simulink subsystem "PowerSystemRef"  (R2024b)
settings: Solver=VariableStepAuto  StartTime=0.0  StopTime=10.0  RelTol=1e-3
undefined symbols (not defined in the file): ess, geom, mot, mot2, mot3, mot4, propel, propel2, propel3, propel4, pxf_diagram_options, SimIn, tc, tc2, tc3, tc4
libraries: simulink x10, slpidlib x5
(part 5 of 10)

== system PowerSystemRef/powerplant/mot4/ctrl/cmd ==
  inport-main_info_bus-1 : Inport
  aInport--2 : Inport  Port=2
  aInport--3 : Inport  Port=3
  aInport--4 : Inport  Port=4
  Terminator_1 : Terminator
  Terminator_2 : Terminator
  Terminator_3 : Terminator
  mot4_ctrl_cmd_map_Pelec_funTW_volt_in : Subsystem
  parameter_out : Subsystem
  parameter_selection : Subsystem
  outport-system_info_bus : Outport
  wires:
  inport-main_info_bus-1/1 -> parameter_selection/1(inport-main_info_bus-1)
  parameter_out/1(outport-system_info_bus) -> outport-system_info_bus/1
  mot4_ctrl_cmd_map_Pelec_funTW_volt_in/1(mot_ctrl_cmd_simu) -> parameter_out/1(inport-mot4_ctrl_cmd_simu)
  parameter_selection/1(outport-mot4_plant_spd_out_simu-1) -> mot4_ctrl_cmd_map_Pelec_funTW_volt_in/1(mot_plant_spd_out_simu)
  parameter_selection/2(outport-mot4_ctrl_trs_trq_simu-2) -> mot4_ctrl_cmd_map_Pelec_funTW_volt_in/2(mot_ctrl_trs_trq_simu)
  parameter_selection/3(outport-mot4_ctrl_cstr_trq_max_pos_simu-3) -> mot4_ctrl_cmd_map_Pelec_funTW_volt_in/3(mot_ctrl_cstr_trq_max_pos_simu)
  parameter_selection/4(outport-mot4_ctrl_cstr_trq_max_neg_simu-4) -> mot4_ctrl_cmd_map_Pelec_funTW_volt_in/4(mot_ctrl_cstr_trq_max_neg_simu)
  aInport--2/1 -> Terminator_1/1
  aInport--3/1 -> Terminator_2/1
  aInport--4/1 -> Terminator_3/1

== system PowerSystemRef/powerplant/mot4/ctrl/cstr ==
  inport-main_info_bus-1 : Inport
  aInport--2 : Inport  Port=2
  aInport--3 : Inport  Port=3
  Terminator_1 : Terminator
  Terminator_2 : Terminator
  mot4_ctrl_cstr_map_Pelec_funTW_volt_in : Subsystem
  parameter_out : Subsystem
  parameter_selection : Subsystem
  outport-system_info_bus : Outport
  outport-cstr_bus : Outport  Port=2
  wires:
  inport-main_info_bus-1/1 -> parameter_selection/1(inport-main_info_bus-1)
  parameter_out/1(outport-system_info_bus) -> outport-system_info_bus/1
  parameter_out/2(outport-cstr_bus) -> outport-cstr_bus/1
  mot4_ctrl_cstr_map_Pelec_funTW_volt_in/1(mot_ctrl_cstr_trq_pk_pos_simu) -> parameter_out/1(inport-mot4_ctrl_cstr_trq_pk_pos_simu)
  mot4_ctrl_cstr_map_Pelec_funTW_volt_in/2(mot_ctrl_cstr_trq_max_pos_simu) -> parameter_out/2(inport-mot4_ctrl_cstr_trq_max_pos_simu)
  mot4_ctrl_cstr_map_Pelec_funTW_volt_in/3(mot_ctrl_cstr_trq_pk_neg_simu) -> parameter_out/3(inport-mot4_ctrl_cstr_trq_pk_neg_simu)
  mot4_ctrl_cstr_map_Pelec_funTW_volt_in/4(mot_ctrl_cstr_trq_max_neg_simu) -> parameter_out/4(inport-mot4_ctrl_cstr_trq_max_neg_simu)
  mot4_ctrl_cstr_map_Pelec_funTW_volt_in/5(mot_ctrl_cstr_trq_cont_pos_simu) -> parameter_out/5(inport-mot4_ctrl_cstr_trq_cont_pos_simu)
  mot4_ctrl_cstr_map_Pelec_funTW_volt_in/6(mot_ctrl_cstr_trq_cont_neg_simu) -> parameter_out/6(inport-mot4_ctrl_cstr_trq_cont_neg_simu)
  mot4_ctrl_cstr_map_Pelec_funTW_volt_in/7(mot_ctrl_cstr_temp_coeff_simu) -> parameter_out/7(inport-mot4_ctrl_cstr_temp_coeff_simu)
  parameter_selection/1(outport-mot4_plant_spd_out_simu-1) -> mot4_ctrl_cstr_map_Pelec_funTW_volt_in/1(mot_plant_spd_out_simu)
  parameter_selection/2(outport-mot4_plant_temp_coeff_simu-2) -> mot4_ctrl_cstr_map_Pelec_funTW_volt_in/2(mot_plant_temp_coeff_simu)
  aInport--2/1 -> Terminator_1/1
  aInport--3/1 -> Terminator_2/1

== system PowerSystemRef/powerplant/mot4/ctrl/dmd ==
  inport-main_info_bus-1 : Inport
  aInport--2 : Inport  Port=2
  Terminator_1 : Terminator
  mot4_ctrl_dmd_uas : Subsystem
  parameter_out : Subsystem
  parameter_selection : Subsystem
  outport-system_info_bus : Outport
  outport-dmd_bus : Outport  Port=2
  wires:
  inport-main_info_bus-1/1 -> parameter_selection/1(inport-main_info_bus-1)
  parameter_out/1(outport-system_info_bus) -> outport-system_info_bus/1
  parameter_out/2(outport-dmd_bus) -> outport-dmd_bus/1
  mot4_ctrl_dmd_uas/1(mot_ctrl_trs_trq_simu) -> parameter_out/1(inport-mot4_ctrl_trs_trq_simu)
  mot4_ctrl_dmd_uas/2(mot_ctrl_ratedpwr_simu) -> parameter_out/2(inport-mot4_ctrl_ratedpwr_simu)
  parameter_selection/1(outport-apc_ctrl_dt4_simu-1) -> mot4_ctrl_dmd_uas/1(apc_ctrl_dt_simu)
  parameter_selection/2(outport-env_plant_density_simu-2) -> mot4_ctrl_dmd_uas/2(env_plant_density_simu)
  parameter_selection/3(outport-ess_ctrl_pwr_max_pro_simu-3) -> mot4_ctrl_dmd_uas/3(ess_ctrl_pwr_max_pro_simu)
  parameter_selection/4(outport-propel4_plant_speed_simu-4) -> mot4_ctrl_dmd_uas/4(propel_plant_speed_simu)
  parameter_selection/5(outport-tc4_plant_spd_in_simu-5) -> mot4_ctrl_dmd_uas/5(tc_plant_spd_in_simu)
  aInport--2/1 -> Terminator_1/1

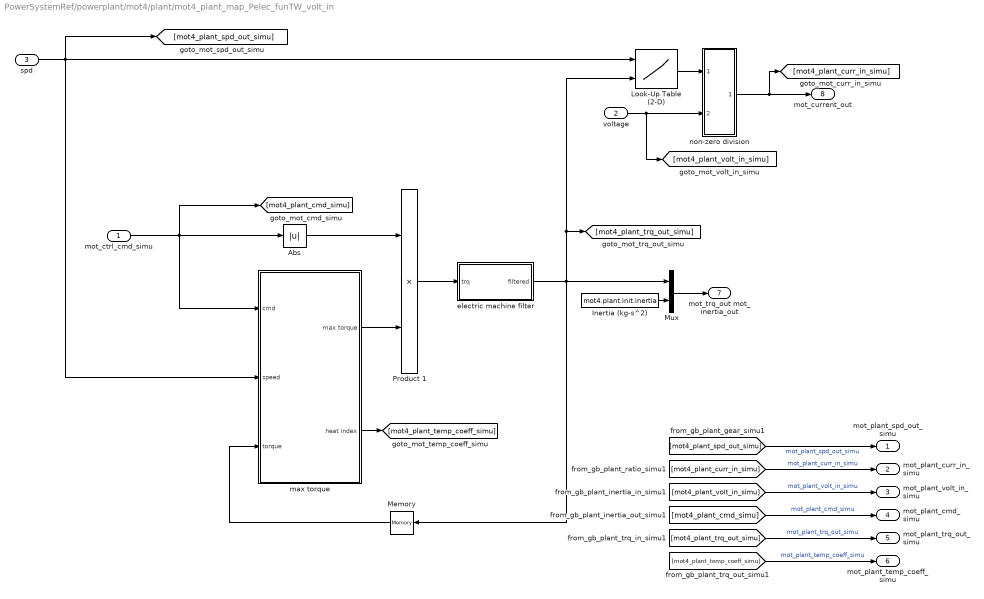
== system PowerSystemRef/powerplant/mot4/plant/mot4_plant_map_Pelec_funTW_volt_in ==
  mot_ctrl_cmd_simu : Inport
  voltage : Inport  Port=2
  spd : Inport  Port=3
  Abs : Abs
  Inertia (kg-s^2) : Constant  Value=mot4.plant.init.inertia
  Look-Up Table (2-D) : Lookup2D  RowIndex=mot4.plant.calc.pwr_elec.idx1_spd  ColumnIndex=mot4.plant.calc.pwr_elec.idx2_trq  Table=mot4.plant.calc.pwr_elec.map
  Memory : Memory
  Mux : Mux  Inputs=2
  Product 1 : Product  InputSameDT=on  SaturateOnIntegerOverflow=on  OutDataTypeStr=Inherit: Same as first input
  electric machine filter : Subsystem
  "max torque " : Subsystem
  non-zero division : Subsystem
      mask Display: disp('divider \n I1/I2')
  mot_plant_spd_out_simu : Outport
  mot_plant_curr_in_simu : Outport  Port=2
  mot_plant_volt_in_simu : Outport  Port=3
  mot_plant_cmd_simu : Outport  Port=4
  mot_plant_trq_out_simu : Outport  Port=5
  mot_plant_temp_coeff_simu : Outport  Port=6
  mot_trq_out mot_inertia_out : Outport  Port=7
  mot_current_out : Outport  Port=8
  wires:
  Look-Up Table (2-D)/1 -> non-zero division/1(In1)
  [mot4_plant_temp_coeff_simu] -> mot_plant_temp_coeff_simu/1  "mot_plant_temp_coeff_simu"
  [mot4_plant_trq_out_simu] -> mot_plant_trq_out_simu/1  "mot_plant_trq_out_simu"
  [mot4_plant_cmd_simu] -> mot_plant_cmd_simu/1  "mot_plant_cmd_simu"
  [mot4_plant_volt_in_simu] -> mot_plant_volt_in_simu/1  "mot_plant_volt_in_simu"
  [mot4_plant_curr_in_simu] -> mot_plant_curr_in_simu/1  "mot_plant_curr_in_simu"
  [mot4_plant_spd_out_simu] -> mot_plant_spd_out_simu/1  "mot_plant_spd_out_simu"
  electric machine filter/1(filtered) -> Mux/1, Memory/1, [mot4_plant_trq_out_simu], Look-Up Table (2-D)/2
  "max torque "/1(max torque) -> Product 1/2
  Product 1/1 -> electric machine filter/1(trq)
  Abs/1 -> Product 1/1
  Memory/1 -> "max torque "/3(torque)
  mot_ctrl_cmd_simu/1 -> "max torque "/1(cmd), [mot4_plant_cmd_simu], Abs/1
  Inertia (kg-s^2)/1 -> Mux/2
  Mux/1 -> mot_trq_out mot_inertia_out/1
  spd/1 -> [mot4_plant_spd_out_simu], "max torque "/2(speed), Look-Up Table (2-D)/1
  "max torque "/2(heat index) -> [mot4_plant_temp_coeff_simu]
  non-zero division/1(Out1) -> mot_current_out/1, [mot4_plant_curr_in_simu]
  voltage/1 -> non-zero division/2(In2), [mot4_plant_volt_in_simu]

== system PowerSystemRef/powerplant/mot4/plant/parameter_out ==
  inport-mot4_plant_spd_out_simu : Inport
  inport-mot4_plant_curr_in_simu : Inport  Port=2
  inport-mot4_plant_volt_in_simu : Inport  Port=3
  inport-mot4_plant_cmd_simu : Inport  Port=4
  inport-mot4_plant_trq_out_simu : Inport  Port=5
  inport-mot4_plant_temp_coeff_simu : Inport  Port=6
  Ground_1 : Ground
  Toworkspace-mot4_plant_cmd_simu : ToWorkspace  VariableName=mot4_plant_cmd_simu  SampleTime=pxf_diagram_options.workspace_sample_time
      settings: Decimation=pxf_diagram_options.decimation
  Toworkspace-mot4_plant_curr_in_simu : ToWorkspace  VariableName=mot4_plant_curr_in_simu  SampleTime=pxf_diagram_options.workspace_sample_time
      settings: Decimation=pxf_diagram_options.decimation
  Toworkspace-mot4_plant_spd_out_simu : ToWorkspace  VariableName=mot4_plant_spd_out_simu  SampleTime=pxf_diagram_options.workspace_sample_time
      settings: Decimation=pxf_diagram_options.decimation
  Toworkspace-mot4_plant_temp_coeff_simu : ToWorkspace  VariableName=mot4_plant_temp_coeff_simu  SampleTime=pxf_diagram_options.workspace_sample_time
      settings: Decimation=pxf_diagram_options.decimation
  Toworkspace-mot4_plant_trq_out_simu : ToWorkspace  VariableName=mot4_plant_trq_out_simu  SampleTime=pxf_diagram_options.workspace_sample_time
      settings: Decimation=pxf_diagram_options.decimation
  Toworkspace-mot4_plant_volt_in_simu : ToWorkspace  VariableName=mot4_plant_volt_in_simu  SampleTime=pxf_diagram_options.workspace_sample_time
      settings: Decimation=pxf_diagram_options.decimation
  create_system_info_bus : BusCreator  Inputs=2
  outport-system_info_bus : Outport
  outport-plant_bus : Outport  Port=2
  wires:
  create_system_info_bus/1 -> outport-system_info_bus/1
  inport-mot4_plant_spd_out_simu/1 -> create_system_info_bus/1, Toworkspace-mot4_plant_spd_out_simu/1  "mot4_plant_spd_out_simu"
  inport-mot4_plant_curr_in_simu/1 -> Toworkspace-mot4_plant_curr_in_simu/1
  inport-mot4_plant_volt_in_simu/1 -> Toworkspace-mot4_plant_volt_in_simu/1
  inport-mot4_plant_cmd_simu/1 -> Toworkspace-mot4_plant_cmd_simu/1
  inport-mot4_plant_trq_out_simu/1 -> Toworkspace-mot4_plant_trq_out_simu/1
  inport-mot4_plant_temp_coeff_simu/1 -> create_system_info_bus/2, Toworkspace-mot4_plant_temp_coeff_simu/1  "mot4_plant_temp_coeff_simu"
  Ground_1/1 -> outport-plant_bus/1

== system PowerSystemRef/powerplant/mot4/plant/parameter_selection ==
  Inport_1 : Inport
  inport-ctrl_bus-2 : Inport  Port=2
  Terminator_1 : Terminator
  select_ctrl_bus : BusSelector  OutputSignals=mot4_ctrl_cmd_simu
  outport-mot4_ctrl_cmd_simu-1 : Outport
  wires:
  inport-ctrl_bus-2/1 -> select_ctrl_bus/1
  select_ctrl_bus/1 -> outport-mot4_ctrl_cmd_simu-1/1  "<mot4_ctrl_cmd_simu>"
  Inport_1/1 -> Terminator_1/1

== system PowerSystemRef/powerplant/propel/plant/parameter_out ==
  inport-propel_plant_speed_simu : Inport
  inport-propel_plant_pwr_in_simu : Inport  Port=2
  inport-propel_plant_pwr_out_simu : Inport  Port=3
  inport-propel_plant_thrust_simu : Inport  Port=4
  Toworkspace-propel_plant_pwr_in_simu : ToWorkspace  VariableName=propel_plant_pwr_in_simu  SampleTime=pxf_diagram_options.workspace_sample_time
      settings: Decimation=pxf_diagram_options.decimation
  Toworkspace-propel_plant_pwr_out_simu : ToWorkspace  VariableName=propel_plant_pwr_out_simu  SampleTime=pxf_diagram_options.workspace_sample_time
      settings: Decimation=pxf_diagram_options.decimation
  Toworkspace-propel_plant_speed_simu : ToWorkspace  VariableName=propel_plant_speed_simu  SampleTime=pxf_diagram_options.workspace_sample_time
      settings: Decimation=pxf_diagram_options.decimation
  Toworkspace-propel_plant_thrust_simu : ToWorkspace  VariableName=propel_plant_thrust_simu  SampleTime=pxf_diagram_options.workspace_sample_time
      settings: Decimation=pxf_diagram_options.decimation
  create_system_info_bus : BusCreator  Inputs=1
  outport-system_info_bus : Outport
  wires:
  create_system_info_bus/1 -> outport-system_info_bus/1
  inport-propel_plant_speed_simu/1 -> create_system_info_bus/1, Toworkspace-propel_plant_speed_simu/1  "propel_plant_speed_simu"
  inport-propel_plant_pwr_in_simu/1 -> Toworkspace-propel_plant_pwr_in_simu/1
  inport-propel_plant_pwr_out_simu/1 -> Toworkspace-propel_plant_pwr_out_simu/1
  inport-propel_plant_thrust_simu/1 -> Toworkspace-propel_plant_thrust_simu/1

== system PowerSystemRef/powerplant/propel/plant/parameter_selection ==
  inport-main_info_bus-1 : Inport
  select_main_info_bus : BusSelector  OutputSignals=env_info_bus.env_plant_density_simu,apa_info_bus.powerplant_info_bus.tc.tc_plant_inertia_out_simu,apa_info_bus.apa_plant_info_bus.apa_plant_info_bus.forceeq_bus.eqnmotion_plant_linvel_simu
  outport-env_plant_density_simu-1 : Outport
  outport-tc_plant_inertia_out_simu-2 : Outport  Port=2
  outport-eqnmotion_plant_linvel_simu-3 : Outport  Port=3
  wires:
  inport-main_info_bus-1/1 -> select_main_info_bus/1
  select_main_info_bus/1 -> outport-env_plant_density_simu-1/1  "<env_plant_density_simu>"
  select_main_info_bus/2 -> outport-tc_plant_inertia_out_simu-2/1  "<tc_plant_inertia_out_simu>"
  select_main_info_bus/3 -> outport-eqnmotion_plant_linvel_simu-3/1  "<eqnmotion_plant_linvel_simu>"

== system PowerSystemRef/powerplant/propel/plant/propel_plant_uas ==
  note: rad/s
  note: rev/s
  env_plant_density_simu : Inport
  tc_plant_inertia_out_simu : Inport  Port=2
  eqnmotion_plant_linvel_simu : Inport  Port=3
  tc_plant_trq_out_simu : Inport  Port=4
  flow-in : Inport  Port=5
  Gain : Gain  Gain=propel.plant.init.thrustdir
  Gain1 : Gain  Gain=2*pi
  Gain2 : Gain
  Gain3 : Gain
  Mux : Mux  Inputs=2
  Propeller Power : Subsystem
  Propeller_CP : Subsystem
  Propeller_Torque : Subsystem
  Terminator : Terminator
  Thrust_Generated : Subsystem
  Total_Moment : Subsystem
  propel_plant_speed_simu : Outport  VectorParamsAs1DForOutWhenUnconnected=off
  propel_plant_pwr_in_simu : Outport  Port=2  VectorParamsAs1DForOutWhenUnconnected=off
  propel_plant_pwr_out_simu : Outport  Port=3  VectorParamsAs1DForOutWhenUnconnected=off
  propel_plant_thrust_simu : Outport  Port=4  VectorParamsAs1DForOutWhenUnconnected=off
  propel_plant_effort : Outport  Port=5  VectorParamsAs1DForOutWhenUnconnected=off
  propel_plant_speed_out_simu : Outport  Port=6  VectorParamsAs1DForOutWhenUnconnected=off
  wires:
  flow-in/1 -> Terminator/1
  Gain3/1 -> propel_plant_speed_simu/1  "propel_plant_speed_simu"
  Gain2/1 -> propel_plant_speed_out_simu/1  "propel_plant_speed_out_simu"
  Propeller Power/1(propel_plant_pwr_in_simu) -> propel_plant_pwr_in_simu/1  "propel_plant_pwr_in_simu"
  Propeller Power/2(propel_plant_pwr_out_simu) -> propel_plant_pwr_out_simu/1  "propel_plant_pwr_out_simu"
  Gain1/1 -> Gain2/1, Gain3/1
  eqnmotion_plant_linvel_simu/1 -> Propeller Power/5(eqnmotion_plant_linvel_simu)
  Mux/1 -> propel_plant_effort/1  "propel_plant_effort"
  Gain/1 -> Mux/1  "effort_plant_longeffort_simu"
  Propeller_Torque/2(propel_plant_restq_simu) -> Total_Moment/2(propel_plant_restq_simu)
  Total_Moment/1(accmoment_plant_totmoment_simu) -> Mux/2  "effort_plant_angleffort_simu"
  tc_plant_inertia_out_simu/1 -> Propeller_Torque/4(tc_plant_inertia_out_simu)
  tc_plant_trq_out_simu/1 -> Propeller_Torque/3(tc_plant_trq_out_simu)
  env_plant_density_simu/1 -> Thrust_Generated/1(env_plant_density_simu), Propeller_Torque/1(env_plant_density_simu)
  Thrust_Generated/2(propel_plant_CT_simu) -> Propeller Power/1(propel_plant_CT_simu)
  Propeller_CP/1(propel_plant_CP_simu) -> Propeller Power/2(propel_plant_CP_simu), Propeller_Torque/2(propel_plant_CP_simu)
  Propeller_Torque/1(propel_plant_rps_simu) -> Propeller Power/4(propel_plant_rps_simu), Gain1/1, Propeller_CP/1(propel_plant_rps_simu), Thrust_Generated/2(propel_plant_speed_simu)
  Thrust_Generated/1(propel_plant_thrust_simu) -> Propeller Power/3(propel_plant_thrust_simu), Total_Moment/1(propel_plant_thrust_simu), Gain/1, propel_plant_thrust_simu/1  "propel_plant_thrust_simu"

== system PowerSystemRef/powerplant/propel2/plant/parameter_out ==
  inport-propel2_plant_speed_simu : Inport
  inport-propel2_plant_pwr_in_simu : Inport  Port=2
  inport-propel2_plant_pwr_out_simu : Inport  Port=3
  inport-propel2_plant_thrust_simu : Inport  Port=4
  Toworkspace-propel2_plant_pwr_in_simu : ToWorkspace  VariableName=propel2_plant_pwr_in_simu  SampleTime=pxf_diagram_options.workspace_sample_time
      settings: Decimation=pxf_diagram_options.decimation
  Toworkspace-propel2_plant_pwr_out_simu : ToWorkspace  VariableName=propel2_plant_pwr_out_simu  SampleTime=pxf_diagram_options.workspace_sample_time
      settings: Decimation=pxf_diagram_options.decimation
  Toworkspace-propel2_plant_speed_simu : ToWorkspace  VariableName=propel2_plant_speed_simu  SampleTime=pxf_diagram_options.workspace_sample_time
      settings: Decimation=pxf_diagram_options.decimation
  Toworkspace-propel2_plant_thrust_simu : ToWorkspace  VariableName=propel2_plant_thrust_simu  SampleTime=pxf_diagram_options.workspace_sample_time
      settings: Decimation=pxf_diagram_options.decimation
  create_system_info_bus : BusCreator  Inputs=1
  outport-system_info_bus : Outport
  wires:
  create_system_info_bus/1 -> outport-system_info_bus/1
  inport-propel2_plant_speed_simu/1 -> create_system_info_bus/1, Toworkspace-propel2_plant_speed_simu/1  "propel2_plant_speed_simu"
  inport-propel2_plant_pwr_in_simu/1 -> Toworkspace-propel2_plant_pwr_in_simu/1
  inport-propel2_plant_pwr_out_simu/1 -> Toworkspace-propel2_plant_pwr_out_simu/1
  inport-propel2_plant_thrust_simu/1 -> Toworkspace-propel2_plant_thrust_simu/1

== system PowerSystemRef/powerplant/propel2/plant/parameter_selection ==
  inport-main_info_bus-1 : Inport
  select_main_info_bus : BusSelector  OutputSignals=env_info_bus.env_plant_density_simu,apa_info_bus.powerplant_info_bus.tc.tc_plant_inertia_out_simu,apa_info_bus.apa_plant_info_bus.apa_plant_info_bus.forceeq_bus.eqnmotion_plant_linvel_simu
  outport-env_plant_density_simu-1 : Outport
  outport-tc_plant_inertia_out_simu-2 : Outport  Port=2
  outport-eqnmotion_plant_linvel_simu-3 : Outport  Port=3
  wires:
  inport-main_info_bus-1/1 -> select_main_info_bus/1
  select_main_info_bus/1 -> outport-env_plant_density_simu-1/1  "<env_plant_density_simu>"
  select_main_info_bus/2 -> outport-tc_plant_inertia_out_simu-2/1  "<tc_plant_inertia_out_simu>"
  select_main_info_bus/3 -> outport-eqnmotion_plant_linvel_simu-3/1  "<eqnmotion_plant_linvel_simu>"

== system PowerSystemRef/powerplant/propel2/plant/propel2_plant_uas ==
  note: rad/s
  note: rev/s
  env_plant_density_simu : Inport
  tc_plant_inertia_out_simu : Inport  Port=2
  eqnmotion_plant_linvel_simu : Inport  Port=3
  tc_plant_trq_out_simu : Inport  Port=4
  flow-in : Inport  Port=5
  Gain : Gain  Gain=propel2.plant.init.thrustdir
  Gain1 : Gain  Gain=2*pi
  Gain2 : Gain
  Gain3 : Gain
  Mux : Mux  Inputs=2
  Propeller Power : Subsystem
  Propeller_CP : Subsystem
  Propeller_Torque : Subsystem
  Terminator : Terminator
  Thrust_Generated : Subsystem
  Total_Moment : Subsystem
  propel_plant_speed_simu : Outport  VectorParamsAs1DForOutWhenUnconnected=off
  propel_plant_pwr_in_simu : Outport  Port=2  VectorParamsAs1DForOutWhenUnconnected=off
  propel_plant_pwr_out_simu : Outport  Port=3  VectorParamsAs1DForOutWhenUnconnected=off
  propel_plant_thrust_simu : Outport  Port=4  VectorParamsAs1DForOutWhenUnconnected=off
  propel_plant_effort : Outport  Port=5  VectorParamsAs1DForOutWhenUnconnected=off
  propel_plant_speed_out_simu : Outport  Port=6  VectorParamsAs1DForOutWhenUnconnected=off
  wires:
  flow-in/1 -> Terminator/1
  Gain3/1 -> propel_plant_speed_simu/1  "propel_plant_speed_simu"
  Gain2/1 -> propel_plant_speed_out_simu/1  "propel_plant_speed_out_simu"
  Propeller Power/1(propel_plant_pwr_in_simu) -> propel_plant_pwr_in_simu/1  "propel_plant_pwr_in_simu"
  Propeller Power/2(propel_plant_pwr_out_simu) -> propel_plant_pwr_out_simu/1  "propel_plant_pwr_out_simu"
  Gain1/1 -> Gain2/1, Gain3/1
  eqnmotion_plant_linvel_simu/1 -> Propeller Power/5(eqnmotion_plant_linvel_simu)
  Mux/1 -> propel_plant_effort/1  "propel_plant_effort"
  Gain/1 -> Mux/1  "effort_plant_longeffort_simu"
  Propeller_Torque/2(propel_plant_restq_simu) -> Total_Moment/2(propel_plant_restq_simu)
  Total_Moment/1(accmoment_plant_totmoment_simu) -> Mux/2  "effort_plant_angleffort_simu"
  tc_plant_inertia_out_simu/1 -> Propeller_Torque/4(tc_plant_inertia_out_simu)
  tc_plant_trq_out_simu/1 -> Propeller_Torque/3(tc_plant_trq_out_simu)
  env_plant_density_simu/1 -> Thrust_Generated/1(env_plant_density_simu), Propeller_Torque/1(env_plant_density_simu)
  Thrust_Generated/2(propel_plant_CT_simu) -> Propeller Power/1(propel_plant_CT_simu)
  Propeller_CP/1(propel_plant_CP_simu) -> Propeller Power/2(propel_plant_CP_simu), Propeller_Torque/2(propel_plant_CP_simu)
  Propeller_Torque/1(propel_plant_rps_simu) -> Propeller Power/4(propel_plant_rps_simu), Gain1/1, Propeller_CP/1(propel_plant_rps_simu), Thrust_Generated/2(propel_plant_speed_simu)
  Thrust_Generated/1(propel_plant_thrust_simu) -> Propeller Power/3(propel_plant_thrust_simu), Total_Moment/1(propel_plant_thrust_simu), Gain/1, propel_plant_thrust_simu/1  "propel_plant_thrust_simu"

== system PowerSystemRef/powerplant/propel3/plant/parameter_out ==
  inport-propel3_plant_speed_simu : Inport
  inport-propel3_plant_pwr_in_simu : Inport  Port=2
  inport-propel3_plant_pwr_out_simu : Inport  Port=3
  inport-propel3_plant_thrust_simu : Inport  Port=4
  Toworkspace-propel3_plant_pwr_in_simu : ToWorkspace  VariableName=propel3_plant_pwr_in_simu  SampleTime=pxf_diagram_options.workspace_sample_time
      settings: Decimation=pxf_diagram_options.decimation
  Toworkspace-propel3_plant_pwr_out_simu : ToWorkspace  VariableName=propel3_plant_pwr_out_simu  SampleTime=pxf_diagram_options.workspace_sample_time
      settings: Decimation=pxf_diagram_options.decimation
  Toworkspace-propel3_plant_speed_simu : ToWorkspace  VariableName=propel3_plant_speed_simu  SampleTime=pxf_diagram_options.workspace_sample_time
      settings: Decimation=pxf_diagram_options.decimation
  Toworkspace-propel3_plant_thrust_simu : ToWorkspace  VariableName=propel3_plant_thrust_simu  SampleTime=pxf_diagram_options.workspace_sample_time
      settings: Decimation=pxf_diagram_options.decimation
  create_system_info_bus : BusCreator  Inputs=1
  outport-system_info_bus : Outport
  wires:
  create_system_info_bus/1 -> outport-system_info_bus/1
  inport-propel3_plant_speed_simu/1 -> create_system_info_bus/1, Toworkspace-propel3_plant_speed_simu/1  "propel3_plant_speed_simu"
  inport-propel3_plant_pwr_in_simu/1 -> Toworkspace-propel3_plant_pwr_in_simu/1
  inport-propel3_plant_pwr_out_simu/1 -> Toworkspace-propel3_plant_pwr_out_simu/1
  inport-propel3_plant_thrust_simu/1 -> Toworkspace-propel3_plant_thrust_simu/1

== system PowerSystemRef/powerplant/propel3/plant/parameter_selection ==
  inport-main_info_bus-1 : Inport
  select_main_info_bus : BusSelector  OutputSignals=env_info_bus.env_plant_density_simu,apa_info_bus.powerplant_info_bus.tc.tc_plant_inertia_out_simu,apa_info_bus.apa_plant_info_bus.apa_plant_info_bus.forceeq_bus.eqnmotion_plant_linvel_simu
  outport-env_plant_density_simu-1 : Outport
  outport-tc_plant_inertia_out_simu-2 : Outport  Port=2
  outport-eqnmotion_plant_linvel_simu-3 : Outport  Port=3
  wires:
  inport-main_info_bus-1/1 -> select_main_info_bus/1
  select_main_info_bus/1 -> outport-env_plant_density_simu-1/1  "<env_plant_density_simu>"
  select_main_info_bus/2 -> outport-tc_plant_inertia_out_simu-2/1  "<tc_plant_inertia_out_simu>"
  select_main_info_bus/3 -> outport-eqnmotion_plant_linvel_simu-3/1  "<eqnmotion_plant_linvel_simu>"

== system PowerSystemRef/powerplant/propel3/plant/propel3_plant_uas ==
  note: rad/s
  note: rev/s
  env_plant_density_simu : Inport
  tc_plant_inertia_out_simu : Inport  Port=2
  eqnmotion_plant_linvel_simu : Inport  Port=3
  tc_plant_trq_out_simu : Inport  Port=4
  flow-in : Inport  Port=5
  Gain : Gain  Gain=propel3.plant.init.thrustdir
  Gain1 : Gain  Gain=2*pi
  Gain2 : Gain
  Gain3 : Gain
  Mux : Mux  Inputs=2
  Propeller Power : Subsystem
  Propeller_CP : Subsystem
  Propeller_Torque : Subsystem
  Terminator : Terminator
  Thrust_Generated : Subsystem
  Total_Moment : Subsystem
  propel_plant_speed_simu : Outport  VectorParamsAs1DForOutWhenUnconnected=off
  propel_plant_pwr_in_simu : Outport  Port=2  VectorParamsAs1DForOutWhenUnconnected=off
  propel_plant_pwr_out_simu : Outport  Port=3  VectorParamsAs1DForOutWhenUnconnected=off
  propel_plant_thrust_simu : Outport  Port=4  VectorParamsAs1DForOutWhenUnconnected=off
  propel_plant_effort : Outport  Port=5  VectorParamsAs1DForOutWhenUnconnected=off
  propel_plant_speed_out_simu : Outport  Port=6  VectorParamsAs1DForOutWhenUnconnected=off
  wires:
  flow-in/1 -> Terminator/1
  Gain3/1 -> propel_plant_speed_simu/1  "propel_plant_speed_simu"
  Gain2/1 -> propel_plant_speed_out_simu/1  "propel_plant_speed_out_simu"
  Propeller Power/1(propel_plant_pwr_in_simu) -> propel_plant_pwr_in_simu/1  "propel_plant_pwr_in_simu"
  Propeller Power/2(propel_plant_pwr_out_simu) -> propel_plant_pwr_out_simu/1  "propel_plant_pwr_out_simu"
  Gain1/1 -> Gain2/1, Gain3/1
  eqnmotion_plant_linvel_simu/1 -> Propeller Power/5(eqnmotion_plant_linvel_simu)
  Mux/1 -> propel_plant_effort/1  "propel_plant_effort"
  Gain/1 -> Mux/1  "effort_plant_longeffort_simu"
  Propeller_Torque/2(propel_plant_restq_simu) -> Total_Moment/2(propel_plant_restq_simu)
  Total_Moment/1(accmoment_plant_totmoment_simu) -> Mux/2  "effort_plant_angleffort_simu"
  tc_plant_inertia_out_simu/1 -> Propeller_Torque/4(tc_plant_inertia_out_simu)
  tc_plant_trq_out_simu/1 -> Propeller_Torque/3(tc_plant_trq_out_simu)
  env_plant_density_simu/1 -> Thrust_Generated/1(env_plant_density_simu), Propeller_Torque/1(env_plant_density_simu)
  Thrust_Generated/2(propel_plant_CT_simu) -> Propeller Power/1(propel_plant_CT_simu)
  Propeller_CP/1(propel_plant_CP_simu) -> Propeller Power/2(propel_plant_CP_simu), Propeller_Torque/2(propel_plant_CP_simu)
  Propeller_Torque/1(propel_plant_rps_simu) -> Propeller Power/4(propel_plant_rps_simu), Gain1/1, Propeller_CP/1(propel_plant_rps_simu), Thrust_Generated/2(propel_plant_speed_simu)
  Thrust_Generated/1(propel_plant_thrust_simu) -> Propeller Power/3(propel_plant_thrust_simu), Total_Moment/1(propel_plant_thrust_simu), Gain/1, propel_plant_thrust_simu/1  "propel_plant_thrust_simu"

== system PowerSystemRef/powerplant/propel4/plant/parameter_out ==
  inport-propel4_plant_speed_simu : Inport
  inport-propel4_plant_pwr_in_simu : Inport  Port=2
  inport-propel4_plant_pwr_out_simu : Inport  Port=3
  inport-propel4_plant_thrust_simu : Inport  Port=4
  Toworkspace-propel4_plant_pwr_in_simu : ToWorkspace  VariableName=propel4_plant_pwr_in_simu  SampleTime=pxf_diagram_options.workspace_sample_time
      settings: Decimation=pxf_diagram_options.decimation
  Toworkspace-propel4_plant_pwr_out_simu : ToWorkspace  VariableName=propel4_plant_pwr_out_simu  SampleTime=pxf_diagram_options.workspace_sample_time
      settings: Decimation=pxf_diagram_options.decimation
  Toworkspace-propel4_plant_speed_simu : ToWorkspace  VariableName=propel4_plant_speed_simu  SampleTime=pxf_diagram_options.workspace_sample_time
      settings: Decimation=pxf_diagram_options.decimation
  Toworkspace-propel4_plant_thrust_simu : ToWorkspace  VariableName=propel4_plant_thrust_simu  SampleTime=pxf_diagram_options.workspace_sample_time
      settings: Decimation=pxf_diagram_options.decimation
  create_system_info_bus : BusCreator  Inputs=1
  outport-system_info_bus : Outport
  wires:
  create_system_info_bus/1 -> outport-system_info_bus/1
  inport-propel4_plant_speed_simu/1 -> create_system_info_bus/1, Toworkspace-propel4_plant_speed_simu/1  "propel4_plant_speed_simu"
  inport-propel4_plant_pwr_in_simu/1 -> Toworkspace-propel4_plant_pwr_in_simu/1
  inport-propel4_plant_pwr_out_simu/1 -> Toworkspace-propel4_plant_pwr_out_simu/1
  inport-propel4_plant_thrust_simu/1 -> Toworkspace-propel4_plant_thrust_simu/1

== system PowerSystemRef/powerplant/propel4/plant/parameter_selection ==
  inport-main_info_bus-1 : Inport
  select_main_info_bus : BusSelector  OutputSignals=env_info_bus.env_plant_density_simu,apa_info_bus.powerplant_info_bus.tc.tc_plant_inertia_out_simu,apa_info_bus.apa_plant_info_bus.apa_plant_info_bus.forceeq_bus.eqnmotion_plant_linvel_simu
  outport-env_plant_density_simu-1 : Outport
  outport-tc_plant_inertia_out_simu-2 : Outport  Port=2
  outport-eqnmotion_plant_linvel_simu-3 : Outport  Port=3
  wires:
  inport-main_info_bus-1/1 -> select_main_info_bus/1
  select_main_info_bus/1 -> outport-env_plant_density_simu-1/1  "<env_plant_density_simu>"
  select_main_info_bus/2 -> outport-tc_plant_inertia_out_simu-2/1  "<tc_plant_inertia_out_simu>"
  select_main_info_bus/3 -> outport-eqnmotion_plant_linvel_simu-3/1  "<eqnmotion_plant_linvel_simu>"

== system PowerSystemRef/powerplant/propel4/plant/propel4_plant_uas ==
  note: rad/s
  note: rev/s
  env_plant_density_simu : Inport
  tc_plant_inertia_out_simu : Inport  Port=2
  eqnmotion_plant_linvel_simu : Inport  Port=3
  tc_plant_trq_out_simu : Inport  Port=4
  flow-in : Inport  Port=5
  Gain : Gain  Gain=propel4.plant.init.thrustdir
  Gain1 : Gain  Gain=2*pi
  Gain2 : Gain
  Gain3 : Gain
  Mux : Mux  Inputs=2
  Propeller Power : Subsystem
  Propeller_CP : Subsystem
  Propeller_Torque : Subsystem
  Terminator : Terminator
  Thrust_Generated : Subsystem
  Total_Moment : Subsystem
  propel_plant_speed_simu : Outport  VectorParamsAs1DForOutWhenUnconnected=off
  propel_plant_pwr_in_simu : Outport  Port=2  VectorParamsAs1DForOutWhenUnconnected=off
  propel_plant_pwr_out_simu : Outport  Port=3  VectorParamsAs1DForOutWhenUnconnected=off
  propel_plant_thrust_simu : Outport  Port=4  VectorParamsAs1DForOutWhenUnconnected=off
  propel_plant_effort : Outport  Port=5  VectorParamsAs1DForOutWhenUnconnected=off
  propel_plant_speed_out_simu : Outport  Port=6  VectorParamsAs1DForOutWhenUnconnected=off
  wires:
  flow-in/1 -> Terminator/1
  Gain3/1 -> propel_plant_speed_simu/1  "propel_plant_speed_simu"
  Gain2/1 -> propel_plant_speed_out_simu/1  "propel_plant_speed_out_simu"
  Propeller Power/1(propel_plant_pwr_in_simu) -> propel_plant_pwr_in_simu/1  "propel_plant_pwr_in_simu"
  Propeller Power/2(propel_plant_pwr_out_simu) -> propel_plant_pwr_out_simu/1  "propel_plant_pwr_out_simu"
  Gain1/1 -> Gain2/1, Gain3/1
  eqnmotion_plant_linvel_simu/1 -> Propeller Power/5(eqnmotion_plant_linvel_simu)
  Mux/1 -> propel_plant_effort/1  "propel_plant_effort"
  Gain/1 -> Mux/1  "effort_plant_longeffort_simu"
  Propeller_Torque/2(propel_plant_restq_simu) -> Total_Moment/2(propel_plant_restq_simu)
  Total_Moment/1(accmoment_plant_totmoment_simu) -> Mux/2  "effort_plant_angleffort_simu"
  tc_plant_inertia_out_simu/1 -> Propeller_Torque/4(tc_plant_inertia_out_simu)
  tc_plant_trq_out_simu/1 -> Propeller_Torque/3(tc_plant_trq_out_simu)
  env_plant_density_simu/1 -> Thrust_Generated/1(env_plant_density_simu), Propeller_Torque/1(env_plant_density_simu)
  Thrust_Generated/2(propel_plant_CT_simu) -> Propeller Power/1(propel_plant_CT_simu)
  Propeller_CP/1(propel_plant_CP_simu) -> Propeller Power/2(propel_plant_CP_simu), Propeller_Torque/2(propel_plant_CP_simu)
  Propeller_Torque/1(propel_plant_rps_simu) -> Propeller Power/4(propel_plant_rps_simu), Gain1/1, Propeller_CP/1(propel_plant_rps_simu), Thrust_Generated/2(propel_plant_speed_simu)
  Thrust_Generated/1(propel_plant_thrust_simu) -> Propeller Power/3(propel_plant_thrust_simu), Total_Moment/1(propel_plant_thrust_simu), Gain/1, propel_plant_thrust_simu/1  "propel_plant_thrust_simu"

== system PowerSystemRef/powerplant/tc/plant/parameter_out ==
  inport-tc_plant_trq_in_simu : Inport
  inport-tc_plant_trq_out_simu : Inport  Port=2
  inport-tc_plant_spd_in_simu : Inport  Port=3
  inport-tc_plant_spd_out_simu : Inport  Port=4
  inport-tc_plant_inertia_in_simu : Inport  Port=5
  inport-tc_plant_inertia_out_simu : Inport  Port=6
  Toworkspace-tc_plant_inertia_in_simu : ToWorkspace  VariableName=tc_plant_inertia_in_simu  SampleTime=pxf_diagram_options.workspace_sample_time
      settings: Decimation=pxf_diagram_options.decimation
  Toworkspace-tc_plant_inertia_out_simu : ToWorkspace  VariableName=tc_plant_inertia_out_simu  SampleTime=pxf_diagram_options.workspace_sample_time
      settings: Decimation=pxf_diagram_options.decimation
  Toworkspace-tc_plant_spd_in_simu : ToWorkspace  VariableName=tc_plant_spd_in_simu  SampleTime=pxf_diagram_options.workspace_sample_time
      settings: Decimation=pxf_diagram_options.decimation
  Toworkspace-tc_plant_spd_out_simu : ToWorkspace  VariableName=tc_plant_spd_out_simu  SampleTime=pxf_diagram_options.workspace_sample_time
      settings: Decimation=pxf_diagram_options.decimation
  Toworkspace-tc_plant_trq_in_simu : ToWorkspace  VariableName=tc_plant_trq_in_simu  SampleTime=pxf_diagram_options.workspace_sample_time
      settings: Decimation=pxf_diagram_options.decimation
  Toworkspace-tc_plant_trq_out_simu : ToWorkspace  VariableName=tc_plant_trq_out_simu  SampleTime=pxf_diagram_options.workspace_sample_time
      settings: Decimation=pxf_diagram_options.decimation
  create_system_info_bus : BusCreator  Inputs=2
  outport-system_info_bus : Outport
  wires:
  create_system_info_bus/1 -> outport-system_info_bus/1
  inport-tc_plant_trq_in_simu/1 -> Toworkspace-tc_plant_trq_in_simu/1
  inport-tc_plant_trq_out_simu/1 -> Toworkspace-tc_plant_trq_out_simu/1
  inport-tc_plant_spd_in_simu/1 -> create_system_info_bus/1, Toworkspace-tc_plant_spd_in_simu/1  "tc_plant_spd_in_simu"
  inport-tc_plant_spd_out_simu/1 -> Toworkspace-tc_plant_spd_out_simu/1
  inport-tc_plant_inertia_in_simu/1 -> Toworkspace-tc_plant_inertia_in_simu/1
  inport-tc_plant_inertia_out_simu/1 -> create_system_info_bus/2, Toworkspace-tc_plant_inertia_out_simu/1  "tc_plant_inertia_out_simu"

== system PowerSystemRef/powerplant/tc/plant/parameter_selection ==

== system PowerSystemRef/powerplant/tc/plant/tc_plant_map_trqloss_funTW ==
  tc_trq_in tc_inertia_in : Inport
  tc_spd_out : Inport  Port=2
  Demux : Demux  Outputs=2
  Inertia calculation : Subsystem
  Mux1 : Mux  Inputs=2
  Speed calculation : Subsystem
  Torque calculation : Subsystem
  tc_plant_trq_in_simu : Outport
  tc_plant_trq_out_simu : Outport  Port=2
  tc_plant_spd_in_simu : Outport  Port=3
  tc_plant_spd_out_simu : Outport  Port=4
  tc_plant_inertia_in_simu : Outport  Port=5
  tc_plant_inertia_out_simu : Outport  Port=6
  tc_trq_out : Outport  Port=7
  tc_spd_in : Outport  Port=8
  wires:
  tc_trq_in tc_inertia_in/1 -> Demux/1
  Mux1/1 -> tc_trq_out/1
  [tc_plant_trq_in_simu] -> tc_plant_trq_in_simu/1  "tc_plant_trq_in_simu"
  [tc_plant_trq_out_simu] -> tc_plant_trq_out_simu/1  "tc_plant_trq_out_simu"
  [tc_plant_spd_in_simu] -> tc_plant_spd_in_simu/1  "tc_plant_spd_in_simu"
  [tc_plant_spd_out_simu] -> tc_plant_spd_out_simu/1  "tc_plant_spd_out_simu"
  [tc_plant_inertia_in_simu] -> tc_plant_inertia_in_simu/1  "tc_plant_inertia_in_simu"
  [tc_plant_inertia_out_simu] -> tc_plant_inertia_out_simu/1  "tc_plant_inertia_out_simu"
  Torque calculation/1(trq out) -> [tc_plant_trq_out_simu], Mux1/1  "tc_plant_trq_out_simu"
  Inertia calculation/1(inertia out) -> [tc_plant_inertia_out_simu], Mux1/2  "tc_plant_inertia_out_simu"
  Demux/2 -> [tc_plant_inertia_in_simu], Inertia calculation/1(inertia in)
  Demux/1 -> Torque calculation/2(trq in), [tc_plant_trq_in_simu]
  tc_spd_out/1 -> [tc_plant_spd_out_simu], Speed calculation/1(spd out)
  Speed calculation/1(spd in) -> Torque calculation/1(spd in), [tc_plant_spd_in_simu], tc_spd_in/1

== system PowerSystemRef/powerplant/tc2/plant/parameter_out ==
  inport-tc2_plant_trq_in_simu : Inport
  inport-tc2_plant_trq_out_simu : Inport  Port=2
  inport-tc2_plant_spd_in_simu : Inport  Port=3
  inport-tc2_plant_spd_out_simu : Inport  Port=4
  inport-tc2_plant_inertia_in_simu : Inport  Port=5
  inport-tc2_plant_inertia_out_simu : Inport  Port=6
  Toworkspace-tc2_plant_inertia_in_simu : ToWorkspace  VariableName=tc2_plant_inertia_in_simu  SampleTime=pxf_diagram_options.workspace_sample_time
      settings: Decimation=pxf_diagram_options.decimation
  Toworkspace-tc2_plant_inertia_out_simu : ToWorkspace  VariableName=tc2_plant_inertia_out_simu  SampleTime=pxf_diagram_options.workspace_sample_time
      settings: Decimation=pxf_diagram_options.decimation
  Toworkspace-tc2_plant_spd_in_simu : ToWorkspace  VariableName=tc2_plant_spd_in_simu  SampleTime=pxf_diagram_options.workspace_sample_time
      settings: Decimation=pxf_diagram_options.decimation
  Toworkspace-tc2_plant_spd_out_simu : ToWorkspace  VariableName=tc2_plant_spd_out_simu  SampleTime=pxf_diagram_options.workspace_sample_time
      settings: Decimation=pxf_diagram_options.decimation
  Toworkspace-tc2_plant_trq_in_simu : ToWorkspace  VariableName=tc2_plant_trq_in_simu  SampleTime=pxf_diagram_options.workspace_sample_time
      settings: Decimation=pxf_diagram_options.decimation
  Toworkspace-tc2_plant_trq_out_simu : ToWorkspace  VariableName=tc2_plant_trq_out_simu  SampleTime=pxf_diagram_options.workspace_sample_time
      settings: Decimation=pxf_diagram_options.decimation
  create_system_info_bus : BusCreator  Inputs=1
  outport-system_info_bus : Outport
  wires:
  create_system_info_bus/1 -> outport-system_info_bus/1
  inport-tc2_plant_trq_in_simu/1 -> Toworkspace-tc2_plant_trq_in_simu/1
  inport-tc2_plant_trq_out_simu/1 -> Toworkspace-tc2_plant_trq_out_simu/1
  inport-tc2_plant_spd_in_simu/1 -> create_system_info_bus/1, Toworkspace-tc2_plant_spd_in_simu/1  "tc2_plant_spd_in_simu"
  inport-tc2_plant_spd_out_simu/1 -> Toworkspace-tc2_plant_spd_out_simu/1
  inport-tc2_plant_inertia_in_simu/1 -> Toworkspace-tc2_plant_inertia_in_simu/1
  inport-tc2_plant_inertia_out_simu/1 -> Toworkspace-tc2_plant_inertia_out_simu/1

== system PowerSystemRef/powerplant/tc2/plant/parameter_selection ==

== system PowerSystemRef/powerplant/tc2/plant/tc2_plant_map_trqloss_funTW ==
  tc_trq_in tc_inertia_in : Inport
  tc_spd_out : Inport  Port=2
  Demux : Demux  Outputs=2
  Inertia calculation : Subsystem
  Mux1 : Mux  Inputs=2
  Speed calculation : Subsystem
  Torque calculation : Subsystem
  tc_plant_trq_in_simu : Outport
  tc_plant_trq_out_simu : Outport  Port=2
  tc_plant_spd_in_simu : Outport  Port=3
  tc_plant_spd_out_simu : Outport  Port=4
  tc_plant_inertia_in_simu : Outport  Port=5
  tc_plant_inertia_out_simu : Outport  Port=6
  tc_trq_out : Outport  Port=7
  tc_spd_in : Outport  Port=8
  wires:
  tc_trq_in tc_inertia_in/1 -> Demux/1
  Mux1/1 -> tc_trq_out/1
  [tc2_plant_trq_in_simu] -> tc_plant_trq_in_simu/1  "tc_plant_trq_in_simu"
  [tc2_plant_trq_out_simu] -> tc_plant_trq_out_simu/1  "tc_plant_trq_out_simu"
  [tc2_plant_spd_in_simu] -> tc_plant_spd_in_simu/1  "tc_plant_spd_in_simu"
  [tc2_plant_spd_out_simu] -> tc_plant_spd_out_simu/1  "tc_plant_spd_out_simu"
  [tc2_plant_inertia_in_simu] -> tc_plant_inertia_in_simu/1  "tc_plant_inertia_in_simu"
  [tc2_plant_inertia_out_simu] -> tc_plant_inertia_out_simu/1  "tc_plant_inertia_out_simu"
  Torque calculation/1(trq out) -> [tc2_plant_trq_out_simu], Mux1/1  "tc_plant_trq_out_simu"
  Inertia calculation/1(inertia out) -> [tc2_plant_inertia_out_simu], Mux1/2  "tc_plant_inertia_out_simu"
  Demux/2 -> [tc2_plant_inertia_in_simu], Inertia calculation/1(inertia in)
  Demux/1 -> Torque calculation/2(trq in), [tc2_plant_trq_in_simu]
  tc_spd_out/1 -> [tc2_plant_spd_out_simu], Speed calculation/1(spd out)
  Speed calculation/1(spd in) -> Torque calculation/1(spd in), [tc2_plant_spd_in_simu], tc_spd_in/1

== system PowerSystemRef/powerplant/tc3/plant/parameter_out ==
  inport-tc3_plant_trq_in_simu : Inport
  inport-tc3_plant_trq_out_simu : Inport  Port=2
  inport-tc3_plant_spd_in_simu : Inport  Port=3
  inport-tc3_plant_spd_out_simu : Inport  Port=4
  inport-tc3_plant_inertia_in_simu : Inport  Port=5
  inport-tc3_plant_inertia_out_simu : Inport  Port=6
  Toworkspace-tc3_plant_inertia_in_simu : ToWorkspace  VariableName=tc3_plant_inertia_in_simu  SampleTime=pxf_diagram_options.workspace_sample_time
      settings: Decimation=pxf_diagram_options.decimation
  Toworkspace-tc3_plant_inertia_out_simu : ToWorkspace  VariableName=tc3_plant_inertia_out_simu  SampleTime=pxf_diagram_options.workspace_sample_time
      settings: Decimation=pxf_diagram_options.decimation
  Toworkspace-tc3_plant_spd_in_simu : ToWorkspace  VariableName=tc3_plant_spd_in_simu  SampleTime=pxf_diagram_options.workspace_sample_time
      settings: Decimation=pxf_diagram_options.decimation
  Toworkspace-tc3_plant_spd_out_simu : ToWorkspace  VariableName=tc3_plant_spd_out_simu  SampleTime=pxf_diagram_options.workspace_sample_time
      settings: Decimation=pxf_diagram_options.decimation
  Toworkspace-tc3_plant_trq_in_simu : ToWorkspace  VariableName=tc3_plant_trq_in_simu  SampleTime=pxf_diagram_options.workspace_sample_time
      settings: Decimation=pxf_diagram_options.decimation
  Toworkspace-tc3_plant_trq_out_simu : ToWorkspace  VariableName=tc3_plant_trq_out_simu  SampleTime=pxf_diagram_options.workspace_sample_time
      settings: Decimation=pxf_diagram_options.decimation
  create_system_info_bus : BusCreator  Inputs=1
  outport-system_info_bus : Outport
  wires:
  create_system_info_bus/1 -> outport-system_info_bus/1
  inport-tc3_plant_trq_in_simu/1 -> Toworkspace-tc3_plant_trq_in_simu/1
  inport-tc3_plant_trq_out_simu/1 -> Toworkspace-tc3_plant_trq_out_simu/1
  inport-tc3_plant_spd_in_simu/1 -> create_system_info_bus/1, Toworkspace-tc3_plant_spd_in_simu/1  "tc3_plant_spd_in_simu"
  inport-tc3_plant_spd_out_simu/1 -> Toworkspace-tc3_plant_spd_out_simu/1
  inport-tc3_plant_inertia_in_simu/1 -> Toworkspace-tc3_plant_inertia_in_simu/1
  inport-tc3_plant_inertia_out_simu/1 -> Toworkspace-tc3_plant_inertia_out_simu/1

== system PowerSystemRef/powerplant/tc3/plant/parameter_selection ==

== system PowerSystemRef/powerplant/tc3/plant/tc3_plant_map_trqloss_funTW ==
  tc_trq_in tc_inertia_in : Inport
  tc_spd_out : Inport  Port=2
  Demux : Demux  Outputs=2
  Inertia calculation : Subsystem
  Mux1 : Mux  Inputs=2
  Speed calculation : Subsystem
  Torque calculation : Subsystem
  tc_plant_trq_in_simu : Outport
  tc_plant_trq_out_simu : Outport  Port=2
  tc_plant_spd_in_simu : Outport  Port=3
  tc_plant_spd_out_simu : Outport  Port=4
  tc_plant_inertia_in_simu : Outport  Port=5
  tc_plant_inertia_out_simu : Outport  Port=6
  tc_trq_out : Outport  Port=7
  tc_spd_in : Outport  Port=8
  wires:
  tc_trq_in tc_inertia_in/1 -> Demux/1
  Mux1/1 -> tc_trq_out/1
  [tc3_plant_trq_in_simu] -> tc_plant_trq_in_simu/1  "tc_plant_trq_in_simu"
  [tc3_plant_trq_out_simu] -> tc_plant_trq_out_simu/1  "tc_plant_trq_out_simu"
  [tc3_plant_spd_in_simu] -> tc_plant_spd_in_simu/1  "tc_plant_spd_in_simu"
  [tc3_plant_spd_out_simu] -> tc_plant_spd_out_simu/1  "tc_plant_spd_out_simu"
  [tc3_plant_inertia_in_simu] -> tc_plant_inertia_in_simu/1  "tc_plant_inertia_in_simu"
  [tc3_plant_inertia_out_simu] -> tc_plant_inertia_out_simu/1  "tc_plant_inertia_out_simu"
  Torque calculation/1(trq out) -> [tc3_plant_trq_out_simu], Mux1/1  "tc_plant_trq_out_simu"
  Inertia calculation/1(inertia out) -> [tc3_plant_inertia_out_simu], Mux1/2  "tc_plant_inertia_out_simu"
  Demux/2 -> [tc3_plant_inertia_in_simu], Inertia calculation/1(inertia in)
  Demux/1 -> Torque calculation/2(trq in), [tc3_plant_trq_in_simu]
  tc_spd_out/1 -> [tc3_plant_spd_out_simu], Speed calculation/1(spd out)
  Speed calculation/1(spd in) -> Torque calculation/1(spd in), [tc3_plant_spd_in_simu], tc_spd_in/1

== system PowerSystemRef/powerplant/tc4/plant/parameter_out ==
  inport-tc4_plant_trq_in_simu : Inport
  inport-tc4_plant_trq_out_simu : Inport  Port=2
  inport-tc4_plant_spd_in_simu : Inport  Port=3
  inport-tc4_plant_spd_out_simu : Inport  Port=4
  inport-tc4_plant_inertia_in_simu : Inport  Port=5
  inport-tc4_plant_inertia_out_simu : Inport  Port=6
  Toworkspace-tc4_plant_inertia_in_simu : ToWorkspace  VariableName=tc4_plant_inertia_in_simu  SampleTime=pxf_diagram_options.workspace_sample_time
      settings: Decimation=pxf_diagram_options.decimation
  Toworkspace-tc4_plant_inertia_out_simu : ToWorkspace  VariableName=tc4_plant_inertia_out_simu  SampleTime=pxf_diagram_options.workspace_sample_time
      settings: Decimation=pxf_diagram_options.decimation
  Toworkspace-tc4_plant_spd_in_simu : ToWorkspace  VariableName=tc4_plant_spd_in_simu  SampleTime=pxf_diagram_options.workspace_sample_time
      settings: Decimation=pxf_diagram_options.decimation
  Toworkspace-tc4_plant_spd_out_simu : ToWorkspace  VariableName=tc4_plant_spd_out_simu  SampleTime=pxf_diagram_options.workspace_sample_time
      settings: Decimation=pxf_diagram_options.decimation
  Toworkspace-tc4_plant_trq_in_simu : ToWorkspace  VariableName=tc4_plant_trq_in_simu  SampleTime=pxf_diagram_options.workspace_sample_time
      settings: Decimation=pxf_diagram_options.decimation
  Toworkspace-tc4_plant_trq_out_simu : ToWorkspace  VariableName=tc4_plant_trq_out_simu  SampleTime=pxf_diagram_options.workspace_sample_time
      settings: Decimation=pxf_diagram_options.decimation
  create_system_info_bus : BusCreator  Inputs=1
  outport-system_info_bus : Outport
  wires:
  create_system_info_bus/1 -> outport-system_info_bus/1
  inport-tc4_plant_trq_in_simu/1 -> Toworkspace-tc4_plant_trq_in_simu/1
  inport-tc4_plant_trq_out_simu/1 -> Toworkspace-tc4_plant_trq_out_simu/1
  inport-tc4_plant_spd_in_simu/1 -> create_system_info_bus/1, Toworkspace-tc4_plant_spd_in_simu/1  "tc4_plant_spd_in_simu"
  inport-tc4_plant_spd_out_simu/1 -> Toworkspace-tc4_plant_spd_out_simu/1
  inport-tc4_plant_inertia_in_simu/1 -> Toworkspace-tc4_plant_inertia_in_simu/1
  inport-tc4_plant_inertia_out_simu/1 -> Toworkspace-tc4_plant_inertia_out_simu/1

== system PowerSystemRef/powerplant/tc4/plant/parameter_selection ==

== system PowerSystemRef/powerplant/tc4/plant/tc4_plant_map_trqloss_funTW ==
  tc_trq_in tc_inertia_in : Inport
  tc_spd_out : Inport  Port=2
  Demux : Demux  Outputs=2
  Inertia calculation : Subsystem
  Mux1 : Mux  Inputs=2
  Speed calculation : Subsystem
  Torque calculation : Subsystem
  tc_plant_trq_in_simu : Outport
  tc_plant_trq_out_simu : Outport  Port=2
  tc_plant_spd_in_simu : Outport  Port=3
  tc_plant_spd_out_simu : Outport  Port=4
  tc_plant_inertia_in_simu : Outport  Port=5
  tc_plant_inertia_out_simu : Outport  Port=6
  tc_trq_out : Outport  Port=7
  tc_spd_in : Outport  Port=8
  wires:
  tc_trq_in tc_inertia_in/1 -> Demux/1
  Mux1/1 -> tc_trq_out/1
  [tc4_plant_trq_in_simu] -> tc_plant_trq_in_simu/1  "tc_plant_trq_in_simu"
  [tc4_plant_trq_out_simu] -> tc_plant_trq_out_simu/1  "tc_plant_trq_out_simu"
  [tc4_plant_spd_in_simu] -> tc_plant_spd_in_simu/1  "tc_plant_spd_in_simu"
  [tc4_plant_spd_out_simu] -> tc_plant_spd_out_simu/1  "tc_plant_spd_out_simu"
  [tc4_plant_inertia_in_simu] -> tc_plant_inertia_in_simu/1  "tc_plant_inertia_in_simu"
  [tc4_plant_inertia_out_simu] -> tc_plant_inertia_out_simu/1  "tc_plant_inertia_out_simu"
  Torque calculation/1(trq out) -> [tc4_plant_trq_out_simu], Mux1/1  "tc_plant_trq_out_simu"
  Inertia calculation/1(inertia out) -> [tc4_plant_inertia_out_simu], Mux1/2  "tc_plant_inertia_out_simu"
  Demux/2 -> [tc4_plant_inertia_in_simu], Inertia calculation/1(inertia in)
  Demux/1 -> Torque calculation/2(trq in), [tc4_plant_trq_in_simu]
  tc_spd_out/1 -> [tc4_plant_spd_out_simu], Speed calculation/1(spd out)
  Speed calculation/1(spd in) -> Torque calculation/1(spd in), [tc4_plant_spd_in_simu], tc_spd_in/1

== system PowerSystemRef/propel/plant/propel_plant_uas/Propeller Power ==
  propel_plant_CT_simu : Inport
  propel_plant_CP_simu : Inport  Port=2
  propel_plant_thrust_simu : Inport  Port=3
  propel_plant_rps_simu : Inport  Port=4
  eqnmotion_plant_linvel_simu : Inport  Port=5
  Dot Product : DotProduct  OutDataTypeStr=Inherit: Inherit via internal rule
  Fcn : Fcn  Expr=u(2) / u(1) * u(4) * u(3) * propel.plant.init.propD
  Mux : Mux
  Product : Product
  Sqrt : Sqrt
  propel_plant_pwr_in_simu : Outport  VectorParamsAs1DForOutWhenUnconnected=off
  propel_plant_pwr_out_simu : Outport  Port=2  VectorParamsAs1DForOutWhenUnconnected=off
  wires:
  Dot Product/1 -> Sqrt/1
  eqnmotion_plant_linvel_simu/1 -> Dot Product/1, Dot Product/2
  Sqrt/1 -> Product/2  "tas"
  Product/1 -> propel_plant_pwr_out_simu/1
  Mux/1 -> Fcn/1
  propel_plant_CT_simu/1 -> Mux/1
  propel_plant_thrust_simu/1 -> Mux/3, Product/1
  propel_plant_rps_simu/1 -> Mux/4
  Fcn/1 -> propel_plant_pwr_in_simu/1  "propel_plant_pwr_in_simu"
  propel_plant_CP_simu/1 -> Mux/2

== system PowerSystemRef/propel/plant/propel_plant_uas/Propeller_CP ==
  propel_plant_rps_simu : Inport
  propel_plant_init_CP_CT_map : Subsystem  mask{x=propel.plant.init.CP_CT_map(:,1)/60, map=propel.plant.init.CP_CT_map(:,3)}
  propel_plant_CP_simu : Outport  VectorParamsAs1DForOutWhenUnconnected=off
  wires:
  propel_plant_init_CP_CT_map/1(output) -> propel_plant_CP_simu/1
  propel_plant_rps_simu/1 -> propel_plant_init_CP_CT_map/1(input x)

== system PowerSystemRef/propel/plant/propel_plant_uas/Propeller_Torque ==
  note: I = Wprop*R^2/3g
      | General Aviation Aircraft Design pg 619
  env_plant_density_simu : Inport
  propel_plant_CP_simu : Inport  Port=2
  tc_plant_trq_out_simu : Inport  Port=3
  tc_plant_inertia_out_simu : Inport  Port=4
  " " : Gain  Gain=-1
  "2pi " : Gain  Gain=1/2/pi
  Demux : Demux  Outputs=2
  Fcn1 : Fcn  Expr=(u(1)/(2*pi)) *u(3)*(u(2)^2)*(propel.plant.init.propD^5)
  Integrator1 : Integrator  InitialCondition=propel.ctrl.init.rps
  Mux : Mux  Inputs=3
  Product : Product  Inputs=*/
  Prop Inertia : Constant  Value=propel.plant.init.Iprop
  Sum1 : Sum  Inputs=|+-
  Sum2 : Sum  Inputs=|++
  Terminator : Terminator
  propel_plant_rps_simu : Outport  VectorParamsAs1DForOutWhenUnconnected=off
  propel_plant_restq_simu : Outport  Port=2  VectorParamsAs1DForOutWhenUnconnected=off
  wires:
  Demux/2 -> Terminator/1
  Demux/1 -> Sum1/1
  "2pi "/1 -> Integrator1/1
  Mux/1 -> Fcn1/1
  " "/1 -> propel_plant_restq_simu/1
  Integrator1/1 -> propel_plant_rps_simu/1, Mux/2  "propeller_plant_rps_simu"
  env_plant_density_simu/1 -> Mux/3  "env_plant_density_simu"
  propel_plant_CP_simu/1 -> Mux/1  "prop_plant_CP_simu"
  tc_plant_trq_out_simu/1 -> Demux/1
  Fcn1/1 -> Sum1/2, " "/1  "propel_plant_restq_simu"
  Prop Inertia/1 -> Sum2/1
  tc_plant_inertia_out_simu/1 -> Sum2/2
  Sum2/1 -> Product/2
  Sum1/1 -> Product/1
  Product/1 -> "2pi "/1
